simulink library "pedal_wheel_animation_lib"  (Simulink 4.00)
settings Model: LastModifiedBy=bsaunder

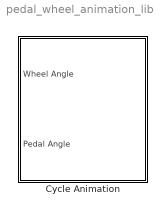
== system pedal_wheel_animation_lib ==
  Cycle Animation : Subsystem  mask{show=on, Ts=0.05}
      mask prompts: show "Show the animation window"; Ts "Sample time"
      mask help: This block provides a visualisation of the cycling action, stimulation pattern and stimulation activation as well as providing read outs of the angle, angular velocity, throttle value and stimulation value.
      settings: RTWFcnNameOpts=Auto  RTWFileNameOpts=Auto
      mask Display:
      | port_label('input', 1, 'Wheel Ang. Vel.');
      | port_label('input', 2, 'Pedal Ang. Vel.');
      | 
      | plot([0.2.*sin([0:(pi/10):2*pi])]+0.3, [0.2.*cos([0:(pi/10):2*pi])]+0.5);
      | plot([0.03.*sin([0:(pi/10):2*pi])]+0.3, [0.03.*cos([0:(pi/10):2*pi])]+0.5);
      | plot([0.07.*sin([0:(pi/10):2*pi])]+0.8, [0.07.*cos([0:(pi/10):2*pi])]+0.5);
      | 
      | plot([0.3 0.3; 0.8 0.8], [0.53 0.47; 0.57 0.43])
      | 
      | plot([0.15.*sin(-pi/4)+0.8 0.15.*sin(3*pi/4)+0.8], [0.15.*cos(-pi/4)+0.5 0.15.*cos(3*pi/4)+0.5]);
      | plot([0.15.*sin([-pi/4:(pi/16):0])]+0.8, [0.15.*cos([-pi/4:(pi/16):0])]+0.5);
      | plot([0.15.*sin([3*pi/4:(pi/16):pi])]+0.8, [0.15.*cos([3*pi/4:(pi/16):pi])]+0.5);
      | 
      | plot([0.77 0.8 0.77], [0.67 0.65 0.62]);
      | plot([0.83 0.8 0.83], [0.38 0.35 0.33]);

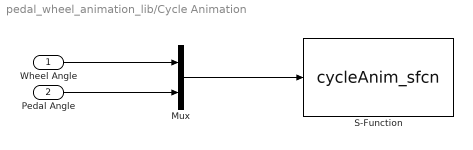
== system pedal_wheel_animation_lib/Cycle Animation ==
  Wheel Angle : Inport  Port=1  LatchInput=off
  Pedal Angle : Inport  Port=2  LatchInput=off
  Mux : Mux  Inputs=2
  S-Function : S-Function  FunctionName=cycleAnim_sfcn  Parameters=Ts, show  PortCounts=[]  SFunctionModules=''
  wires:
  Mux/1 -> S-Function/1
  Wheel Angle/1 -> Mux/1
  Pedal Angle/1 -> Mux/2
